simulink model "SoftStop_Bsp"  (R2015a)
settings: Solver=FixedStepDiscrete  SolverMode=SingleTasking  StartTime=0.0  StopTime=10.0  FixedStep=1e-3  RelTol=1e-3
libraries: mbed_spi_power x5, mbed_lib x4
settings Model: Creator=svenl  LastModifiedBy=oh
settings OptimizationCC: OptimizeModelRefInitCode=on  LifeSpan=1
settings HardwareCC: ProdLargestAtomicInteger=Long  ProdLargestAtomicFloat=Double  ProdEndianess=LittleEndian  ProdHWDeviceType=ARM Compatible->ARM Cortex
settings RTWCC: SystemTargetFile=mbed.tlc  TemplateMakefile=mbed.tmf  Description=Mbed Target (Embedded Target)  TargetLang=C++
settings CodeAppCC: IgnoreCustomStorageClasses=off
settings STFCustomTargetCC: CombineOutputUpdateFcns=on  SupportContinuousTime=off  SupportVariableSizeSignals=off  SystemTargetFile=mbed.tlc
settings ERTTargetCC: SupportContinuousTime=off  SupportVariableSizeSignals=off  ERTCustomFileTemplate=mbed_file_process.tlc

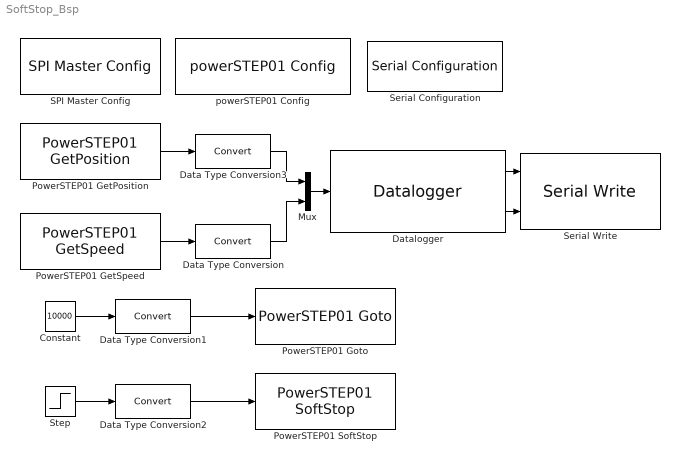
== system SoftStop_Bsp ==
  Constant : Constant  Value=10000
  Data Type Conversion{,1..3} (4 alike) : DataTypeConversion
  Datalogger : mbed_lib/Utilities/Datalogger  TypeInputPorts={ 'double' 2 }  TypeOfInputs={'2*double'}  BufferSize=10000  errEn=off  SampleTime=-1
  Mux : Mux  Inputs=2
  PowerSTEP01 GetPosition : mbed_spi_power/PowerSTEP01 GetPosition  SPINr=1  NumMotors=1  SSELPort=B  SSELPin=6  SampleTime=-1
  PowerSTEP01 GetSpeed : mbed_spi_power/PowerSTEP01 GetSpeed  SPINr=1  NumMotors=1  SSELPort=B  SSELPin=6  SampleTime=-1
  PowerSTEP01 Goto : mbed_spi_power/PowerSTEP01 Goto  SPINr=1  NumMotors=1  SSELPort=B  SSELPin=6  SampleTime=300
  PowerSTEP01 SoftStop : mbed_spi_power/PowerSTEP01 SoftStop  SPINr=1  NumMotors=1  SSELPort=B  SSELPin=6  SampleTime=-1
  SPI Master Config : mbed_lib/SPI/SPI Master Config  Priority=0  SpiPort=1  SpiFreq=100000  MosiPort=A  MosiPin=7  MisoPort=A  MisoPin=6  SclkPort=A  SclkPin=5
  Serial Configuration : mbed_lib/Serial/Serial Configuration  SerialPort=1  TXPort=A  TXPin=2  RXPort=A  RXPin=3  BaudRate=115200
  Serial Write : mbed_lib/Serial/Serial Write  SerialPort=1  numData=on  SampleTime=0.01
  Step : Step  Time=3  SampleTime=0.1
  powerSTEP01 Config : mbed_spi_power/powerSTEP01 Config  Priority=0  SPINr=1  SSELPort=B  SSELPin=6  ResetPort=A  ResetPin=9  ACC=50  DEC=50  MaxSpeed=200  MinSpeed=0  FullStepSpeed=150  Overcurrent=100  StepMode=STEP_MODE_1_128  Holdtorque=20  Runtorque=20  ACCtorque=20  DECtorque=20  Motor2SEL=on  ACC_1=50  DEC_1=50  MaxSpeed_1=500  MinSpeed_1=0  FullStepSpeed_1=350  Overcurrent_1=150  StepMode_1=STEP_MODE_1_32  Holdtorque_1=50  Runtorque_1=50  ACCtorque_1=50  DECtorque_1=50  Motor3SEL=off  ACC_2=0  DEC_2=0  MaxSpeed_2=0  MinSpeed_2=0  FullStepSpeed_2=0  Overcurrent_2=0  StepMode_2=STEP_MODE_FULL  Holdtorque_2=0  Runtorque_2=0  ACCtorque_2=0  DECtorque_2=0
  wires:
  Datalogger/1 -> Serial Write/1
  Datalogger/2 -> Serial Write/2
  Mux/1 -> Datalogger/1
  PowerSTEP01 GetSpeed/1 -> Data Type Conversion/1
  PowerSTEP01 GetPosition/1 -> Data Type Conversion3/1
  Constant/1 -> Data Type Conversion1/1
  Data Type Conversion/1 -> Mux/2
  Data Type Conversion3/1 -> Mux/1
  Data Type Conversion1/1 -> PowerSTEP01 Goto/1
  Step/1 -> Data Type Conversion2/1
  Data Type Conversion2/1 -> PowerSTEP01 SoftStop/1
